simulink model "test_HEx3_mod"  (R2016a)
settings: Solver=ode15s  StartTime=0.0  StopTime=1e5  MaxStep=1e2  RelTol=1e-3
libraries: simCryogenics_lib x26, nesl_utility x26
settings Model: Creator=SK248285  LastModifiedBy=FB229602
settings DataIOCC: LimitDataPoints=on  SaveFormat=Array  SaveState=on
settings HardwareCC: ProdBitPerPointer=32  ProdLargestAtomicFloat=None  ProdIntDivRoundTo=Undefined  ProdEndianess=Unspecified  ProdWordSize=32  ProdHWDeviceType=32-bit Generic
settings ModelReferenceCC: PropagateSignalLabelsOutOfModel=off
settings ConfigComp: CovModelRefEnable=Off
settings SimscapeCC: SimscapeLogType=all  SimscapeLogLimitData=off

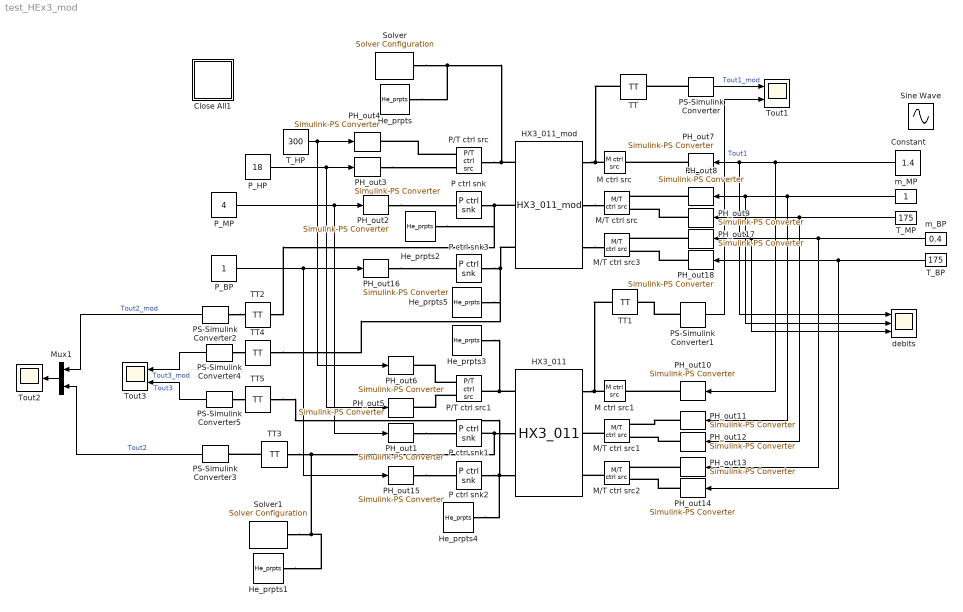
== system test_HEx3_mod ==
  Close All1 : Subsystem
      settings: OpenFcn=|
      | set(0, 'showhiddenhandles', 'on')
      | scope = findobj(0, 'Tag','SIMULINK_SIMSCOPE_FIGURE');
      | close(scope)
      | set(0, 'showhiddenhandles', 'off')
      mask Display: disp('Close\nAll\nScope')
  Constant : Constant  Value=1.4
  HX3_011 : simCryogenics_lib/Elements/HX3_011  N=10  Vh=0.5 m^3  Vm=0.5 m^3  Vc=0.5 m^3  M=1000 kg  Kh=0 s*bar/kg  Km=0 s*bar/kg  Kc=0 s*bar/kg  hh_m=1.4e5 J/s/K  hh_c=0.4e5 J/s/K  hm_c=0 J/s/K  Th0=300 K  Ph0=18 bar  Mh0=1.4 kg/s  Tm0=175 K  Pm0=4 bar  Mm0=1 kg/s  Tc0=175 K  Pc0=1 bar  Mc0=0.4 kg/s  sensh=0  sensm=1  sensc=1
  HX3_011_mod : simCryogenics_lib/Elements_s/HX3_011_mod  N=10  Vh=0.5 m^3  Vm=0.5 m^3  Vc=0.5 m^3  M=1000 kg  Kh=0 s*bar/kg  Km=0 s*bar/kg  Kc=0 s*bar/kg  hn_h=1.8e5 W/K  hn_m=1 W/K  hn_c=0.4 W/K  Th0=300 K  Ph0=18 bar  Mh0=1 kg/s  Tm0=175 K  Pm0=4 bar  Mm0=1 kg/s  Tc0=175 K  Pc0=1 bar  Mc0=1 kg/s  Thn=300 K  Phn=18 bar  Mhn=1 kg/s  Tmn=175 K  Pmn=4 bar  Mmn=1 kg/s  Tcn=175 K  Pcn=1 bar  Mcn=1 kg/s  ex_hp_bp=4  ex_hp_mp=14  ex_mp_bp=0  ex_mode=0  sensh=0  sensm=1  sensc=1
  He_prpts{,1..5} (6 alike) : simCryogenics_lib/Utilities/He_prpts  P_min=0.01 bar  P_max=20 bar  T_min=1.8 K  T_max=400 K  N=100  Mol=4.0026 * 10 ^ (- 3) kg/mol
  M ctrl src : simCryogenics_lib/Sources_Sinks/M ctrl src
  M ctrl src1 : simCryogenics_lib/Sources_Sinks/M ctrl src
  M/T ctrl src{,1..3} (4 alike) : simCryogenics_lib/Sources_Sinks/M//T ctrl src
  Mux1 : Mux  Inputs=2
  P ctrl snk{,1..3} (4 alike) : simCryogenics_lib/Sources_Sinks/P ctrl snk
  P/T ctrl src : simCryogenics_lib/Sources_Sinks/P//T ctrl src
  P/T ctrl src1 : simCryogenics_lib/Sources_Sinks/P//T ctrl src
  PH_out{1..3,5,15..16} (6 alike) : nesl_utility/Simulink-PS Converter  PhysicalDomain=network_engine_domain  SubClassName=ps_input  LeftPortType=input  RightPortType=output  PseudoPeriodic=off  Frequencies=[]  NoiseDistribution=none  NoiseParameters=[]  Unit=bar  AffineConversion=off  InputFiltering=off  SimscapeFilterOrder=1  InputFilterTimeConstant=0.001  UdotUserProvided=1
  PH_out{7..8,10..11,13,17} (6 alike) : nesl_utility/Simulink-PS Converter  PhysicalDomain=network_engine_domain  SubClassName=ps_input  LeftPortType=input  RightPortType=output  PseudoPeriodic=off  Frequencies=[]  NoiseDistribution=none  NoiseParameters=[]  Unit=kg/s  AffineConversion=off  InputFiltering=off  SimscapeFilterOrder=1  InputFilterTimeConstant=0.001  UdotUserProvided=1
  PH_out{4,6,9,12,14,18} (6 alike) : nesl_utility/Simulink-PS Converter  PhysicalDomain=network_engine_domain  SubClassName=ps_input  LeftPortType=input  RightPortType=output  PseudoPeriodic=off  Frequencies=[]  NoiseDistribution=none  NoiseParameters=[]  Unit=K  AffineConversion=off  InputFiltering=off  SimscapeFilterOrder=1  InputFilterTimeConstant=0.001  UdotUserProvided=1
  PS-Simulink Converter{,1..5} (6 alike) : nesl_utility/PS-Simulink Converter  PhysicalDomain=network_engine_domain  SubClassName=ps_output  LeftPortType=input  RightPortType=output  PseudoPeriodic=off  Frequencies=[]  Unit=1  AffineConversion=off
  P_BP : Constant
  P_HP : Constant  Value=18
  P_MP : Constant  Value=4
  Sine Wave : Sin  Bias=1.4  Frequency=1/1e5*2*pi  SampleTime=0
  Solver : nesl_utility/Solver Configuration  PhysicalDomain=network_engine_domain  SubClassName=solver  LeftPortType=input  RightPortType=generic  Accelerate=off  Tones=[]  Harmonics=[]  SimulateNoise=off  Profile=off  UseLocalSampling=off  EnableSwitchedLinearOptims=on  FrequencyDomain=off  UseCCode=off  RelTol=0.001  AbsTol=1e-06  MinStep=1e-09  ToWorkspace=off  RevertToSquareIcSolve=off  NumHomotopyIterations=100  PhasorMode=off  PhasorModeNumHarmonics=1  OverrideAbsTol=off  DoDC=off  ResidualTolerance=1e-2  UseLocalSolver=off  LocalSolverChoice=NE_BACKWARD_EULER_ADVANCER  LocalSolverSampleTime=5  DoFixedCost=off  MaxNonlinIter=3  MaxModeIter=2  LinearAlgebra=Sparse  DelaysMemoryBudget=1024  AutomaticFiltering=on  FilteringTimeConstant=0.001
  Solver1 : nesl_utility/Solver Configuration  PhysicalDomain=network_engine_domain  SubClassName=solver  LeftPortType=input  RightPortType=generic  Accelerate=off  Tones=[]  Harmonics=[]  SimulateNoise=off  Profile=off  UseLocalSampling=off  EnableSwitchedLinearOptims=on  FrequencyDomain=off  UseCCode=off  RelTol=0.001  AbsTol=1e-06  MinStep=1e-09  ToWorkspace=off  RevertToSquareIcSolve=off  NumHomotopyIterations=100  PhasorMode=off  PhasorModeNumHarmonics=1  OverrideAbsTol=off  DoDC=off  ResidualTolerance=1e-02  UseLocalSolver=off  LocalSolverChoice=NE_BACKWARD_EULER_ADVANCER  LocalSolverSampleTime=5  DoFixedCost=off  MaxNonlinIter=3  MaxModeIter=2  LinearAlgebra=Sparse  DelaysMemoryBudget=1024  AutomaticFiltering=on  FilteringTimeConstant=0.001
  TT{,1..5} (6 alike) : simCryogenics_lib/Sensors/TT
  T_BP : Constant  Value=175
  T_HP : Constant  Value=300
  T_MP : Constant  Value=175
  Tout1 : Scope  NumInputPorts=2
  Tout2 : Scope
  Tout3 : Scope  NumInputPorts=2
  debits : Scope  NumInputPorts=3
  m_BP : Constant  Value=0.4
  m_MP : Constant
  wires:
  T_HP/1 -> PH_out6/1, PH_out4/1
  P_MP/1 -> PH_out1/1, PH_out2/1
  P_HP/1 -> PH_out5/1, PH_out3/1
  T_MP/1 -> PH_out12/1, PH_out9/1
  PS-Simulink Converter/1 -> Tout1/1  "Tout1_mod"
  PS-Simulink Converter1/1 -> Tout1/2  "Tout1"
  PS-Simulink Converter2/1 -> Mux1/1  "Tout2_mod"
  Mux1/1 -> Tout2/1
  PS-Simulink Converter3/1 -> Mux1/2  "Tout2"
  Constant/1 -> PH_out7/1, debits/1, PH_out10/1
  m_MP/1 -> PH_out8/1, debits/2, PH_out11/1
  P_BP/1 -> PH_out15/1, PH_out16/1
  m_BP/1 -> PH_out13/1, debits/3, PH_out17/1
  T_BP/1 -> PH_out14/1, PH_out18/1
  PS-Simulink Converter4/1 -> Tout3/1  "Tout3_mod"
  PS-Simulink Converter5/1 -> Tout3/2  "Tout3"
  connections:
  P ctrl snk/RConn1 -- TT2/LConn1 -- He_prpts2/RConn1 -- HX3_011_mod/LConn2
  PH_out3/RConn1 -- P/T ctrl src/LConn1
  PH_out2/RConn1 -- P ctrl snk/LConn1
  P/T ctrl src/LConn2 -- PH_out4/RConn1
  M ctrl src/RConn1 -- HX3_011_mod/RConn3 -- TT/LConn1
  Solver/RConn1 -- P/T ctrl src/RConn1 -- HX3_011_mod/LConn3 -- He_prpts/RConn1
  HX3_011_mod/RConn2 -- M/T ctrl src/RConn1
  He_prpts3/RConn1 -- HX3_011/LConn3 -- P/T ctrl src1/RConn1
  Solver1/RConn1 -- He_prpts1/RConn1 -- HX3_011/LConn2 -- P ctrl snk1/RConn1 -- TT3/LConn1
  M/T ctrl src1/RConn1 -- HX3_011/RConn2
  M ctrl src1/RConn1 -- HX3_011/RConn3 -- TT1/LConn1
  PH_out7/RConn1 -- M ctrl src/LConn1
  PH_out8/RConn1 -- M/T ctrl src/LConn1
  PH_out9/RConn1 -- M/T ctrl src/LConn2
  P/T ctrl src1/LConn2 -- PH_out6/RConn1
  P/T ctrl src1/LConn1 -- PH_out5/RConn1
  PH_out1/RConn1 -- P ctrl snk1/LConn1
  PH_out10/RConn1 -- M ctrl src1/LConn1
  PH_out11/RConn1 -- M/T ctrl src1/LConn1
  PH_out12/RConn1 -- M/T ctrl src1/LConn2
  PS-Simulink Converter/LConn1 -- TT/RConn1
  PS-Simulink Converter1/LConn1 -- TT1/RConn1
  PS-Simulink Converter2/LConn1 -- TT2/RConn1
  TT3/RConn1 -- PS-Simulink Converter3/LConn1
  M/T ctrl src2/RConn1 -- HX3_011/RConn1
  PH_out13/RConn1 -- M/T ctrl src2/LConn1
  PH_out14/RConn1 -- M/T ctrl src2/LConn2
  P ctrl snk2/RConn1 -- He_prpts4/RConn1 -- TT5/LConn1 -- HX3_011/LConn1
  PH_out15/RConn1 -- P ctrl snk2/LConn1
  P ctrl snk3/RConn1 -- HX3_011_mod/LConn1 -- TT4/LConn1 -- He_prpts5/RConn1
  PH_out16/RConn1 -- P ctrl snk3/LConn1
  HX3_011_mod/RConn1 -- M/T ctrl src3/RConn1
  PH_out17/RConn1 -- M/T ctrl src3/LConn1
  PH_out18/RConn1 -- M/T ctrl src3/LConn2
  PS-Simulink Converter4/LConn1 -- TT4/RConn1
  PS-Simulink Converter5/LConn1 -- TT5/RConn1

== system test_HEx3_mod/Close All1 ==
